simulink model "test_rw_to_accel"  (R2022b)
settings: Solver=VariableStepAuto  StartTime=0.0  StopTime=5  FixedStep=1e-5  MaxStep=0.01
settings Model: Creator=Jon  LastModifiedBy=Jon
settings ModelReferenceCC: EnableRefExpFcnMdlSchedulingChecks=on

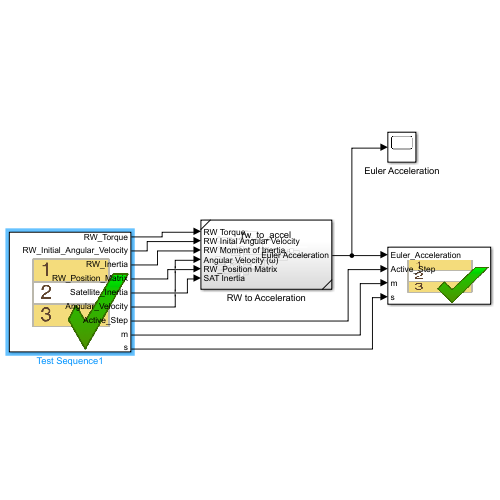
[thumbnail: Simulink's stored preview of the top-level diagram]
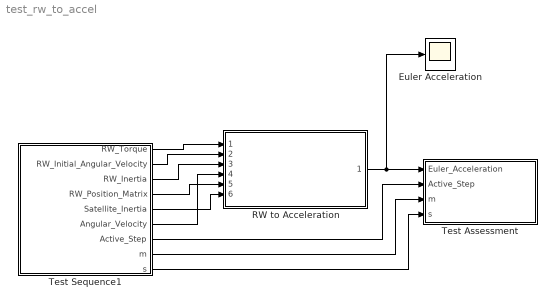
== system test_rw_to_accel ==
  Euler Acceleration : Scope
  RW to Acceleration : Subsystem  ReferencedSubsystem=rw_to_accel
  Test Assessment : Test Sequence  TreatAsAtomicUnit=on
  Test Sequence1 : Test Sequence  TreatAsAtomicUnit=on
  wires:
  RW to Acceleration/1 -> Euler Acceleration/1, Test Assessment/1(Euler_Acceleration)
  Test Sequence1/1(RW_Torque) -> RW to Acceleration/1
  Test Sequence1/2(RW_Initial_Angular_Velocity) -> RW to Acceleration/2
  Test Sequence1/3(RW_Inertia) -> RW to Acceleration/3
  Test Sequence1/4(RW_Position_Matrix) -> RW to Acceleration/5
  Test Sequence1/5(Satellite_Inertia) -> RW to Acceleration/6
  Test Sequence1/6(Angular_Velocity) -> RW to Acceleration/4
  Test Sequence1/7(Active_Step) -> Test Assessment/2(Active_Step)
  Test Sequence1/8(m) -> Test Assessment/3(m)
  Test Sequence1/9(s) -> Test Assessment/4(s)

== stateflow chart test_rw_to_accel/Test Sequence1 ==
  state Test_One
    Transition_Time = 1;
    m = 3; % kg
    s = 0.1; % m
    RW_Inertia = 100.5;
    RW_Position_Matrix = [0; 0; 1];
    RW_Torque = 1;
    RW_Initial_Angular_Velocity = -RW_Torque / RW_Inertia * t;
    Satellite_Inertia = eye(3)*1/6*m*s^2;
    Angular_Velocity = [0; 0; 0];
    settings: description=Test constant torque with no precession
  state Test_Two
    RW_Initial_Angular_Velocity = -RW_Torque / RW_Inertia * t;
    Satellite_Inertia = eye(3)*1/6*m*s^2;
    Angular_Velocity = [2; 0; 0];
    settings: description=Test with initial satellite velocity in one dimension
  state Test_Three
    RW_Initial_Angular_Velocity = -RW_Torque / RW_Inertia * t;
    Satellite_Inertia = eye(3)*1/6*m*s^2;
    Angular_Velocity = [2; 1; 0];
    settings: description=Test with initial satellite velocity in two dimensions
  state Test_Four
    RW_Initial_Angular_Velocity = -RW_Torque / RW_Inertia * t;
    Satellite_Inertia = m*s^2*[[5/12; 0; 0], [0; 5/12; 0], [0; 0; 1/6]];
    Angular_Velocity = [2; 1; 0];
    settings: description=Test with non-cubic satellite
  state Test_Five
    RW_Initial_Angular_Velocity = -RW_Torque / RW_Inertia * t;
    Satellite_Inertia = m*s^2*[[5/12; 0; 0], [0; 5/12; 0], [0; 0; 1/6]];
    Angular_Velocity = [2; 1; 3];
    settings: description=Test with non-cubic satellite and precession
  (default) -> Test_One
  Test_One -> Test_Two : [
      | after(Transition_Time, sec)
      | ]
  Test_Two -> Test_Three : [
      | after(Transition_Time, sec)
      | ]
  Test_Three -> Test_Four : [
      | after(Transition_Time, sec)
      | ]
  Test_Four -> Test_Five : [
      | after(Transition_Time, sec)
      | ]
  data: RW_Torque output; RW_Initial_Angular_Velocity output; RW_Inertia output; RW_Position_Matrix output; Satellite_Inertia output; Angular_Velocity output; Active_Step output Enum: Active_Step_Enum; m output; s output; Transition_Time local

== stateflow chart test_rw_to_accel/Test Assessment ==
  state Initialization
    Tol = 1e-10; % tolerance for results,
  state Assessments
    state Verify_One
      verify(all(abs(Euler_Acceleration - [0; 0; -6/(m*s^2)]) < Tol))
    state Verify_Two
      verify(all(abs(Euler_Acceleration - [0; 0; -6/(m*s^2)]) < Tol))
    state Verify_Three
      verify(all(abs(Euler_Acceleration - [0; 0; -6/(m*s^2)]) < Tol))
    state Verify_Four
      verify(all(abs(Euler_Acceleration - [0; 0; -6/(m*s^2)]) < Tol))
    state Verify_Five
      verify(all(abs(Euler_Acceleration - [63/10; -63/5; -6/(m*s^2)]) < Tol))
    state Else
    (default) -> (junction 85)
    (junction 55) -> Verify_One [order 1] : [~in(Assessments.Verify_One)]
    (junction 85) -> (junction 55) [order 1] : [Active_Step == Active_Step_Enum.Test_One
        | ]
    (junction 55) -> (junction 58) [order 2]
    Assessments -> (junction 85)
    (junction 85) -> (junction 76) [order 2]
    (junction 76) -> (junction 77) [order 1] : [Active_Step == Active_Step_Enum.Test_Two
        | ]
    (junction 77) -> Verify_Two [order 1] : [~in(Assessments.Verify_Two)]
    (junction 76) -> (junction 105) [order 2]
    (junction 77) -> (junction 80) [order 2]
    (junction 105) -> (junction 106) [order 1] : [Active_Step == Active_Step_Enum.Test_Three
        | ]
    (junction 106) -> Verify_Three [order 1] : [~in(Assessments.Verify_Three)]
    (junction 105) -> (junction 126) [order 2]
    (junction 106) -> (junction 109) [order 2]
    (junction 126) -> (junction 127) [order 1] : [Active_Step == Active_Step_Enum.Test_Four
        | ]
    (junction 127) -> Verify_Four [order 1] : [~in(Assessments.Verify_Four)]
    (junction 126) -> (junction 135) [order 2]
    (junction 127) -> (junction 130) [order 2]
    (junction 135) -> (junction 136) [order 1] : [Active_Step == Active_Step_Enum.Test_Five
        | ]
    (junction 136) -> Verify_Five [order 1] : [~in(Assessments.Verify_Five)]
    (junction 135) -> (junction 96) [order 2]
    (junction 136) -> (junction 139) [order 2]
    (junction 96) -> (junction 97)
    (junction 97) -> Else [order 1] : [~in(Assessments.Else)]
    (junction 97) -> (junction 100) [order 2]
  (default) -> Initialization
  Initialization -> Assessments : [
      | true
      | ]
  data: Euler_Acceleration input; Active_Step input; m input; s input; Tol local
